simulink model "ScooterCharacteristic"  (R2024a)
settings: Solver=VariableStepAuto  StartTime=0.0  StopTime=Inf  RelTol=1e-3
libraries: fl_lib x6, nesl_utility x3
settings Model: Creator=vboutrou  LastModifiedBy=vboutrou
settings RTWCC: GPUComputeCapability=3.5
settings SimscapeCC: SimscapeLogType=all

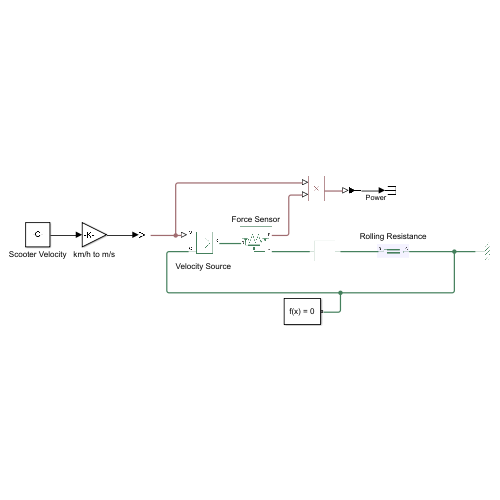
[thumbnail: Simulink's stored preview of the top-level diagram]
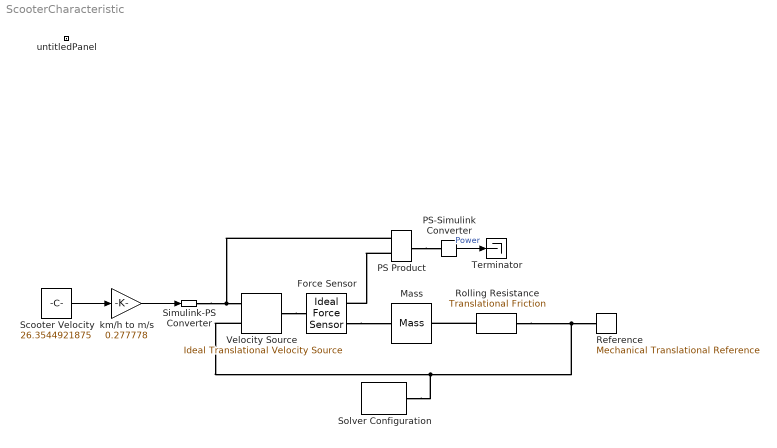
== system ScooterCharacteristic ==
  Force Sensor : fl_lib/Mechanical/Mechanical Sensors/Ideal Force Sensor
  Mass : fl_lib/Mechanical/Translational Elements/Mass  mass=90 kg  num_ports=foundation.enum.numPorts2.two  v_specify=off  v_priority=High  v=0 m/s  v_nominal_specify=off  v_nominal_value=1  v_nominal_unit=m/s  f_specify=off  f_priority=None  f=0 N  f_nominal_specify=off  f_nominal_value=1  f_nominal_unit=N
      settings: InternalSimscapePortConfiguration="{\"Bottom\":[],\"Left\":[{\"id\":\"M\",\"label\":\"\",\"type\":\"foundation.mechanical.translational.translational\"}],\"Right\":[{\"id\":\"N\",\"label\":\"\",\"type\":\"foundation.mechanical.translational.translational\"}],\"Top\":[]}"
  PS Product : fl_lib/Physical Signals/Functions/PS Product
  PS-Simulink Converter : nesl_utility/PS-Simulink Converter  PhysicalDomain=network_engine_domain  SubClassName=ps_output  LeftPortType=input  RightPortType=output  PseudoPeriodic=off  Frequencies=[]  VectorFormat=inherit  Unit=inherit  AffineConversion=off
  Reference : fl_lib/Mechanical/Translational Elements/Mechanical Translational Reference
  Rolling Resistance : fl_lib/Mechanical/Translational Elements/Translational Friction  brkwy_frc=20 N  brkwy_vel=0.1 m/s  Col_frc=14 N  visc_coef=3.1 N/(m/s)  v_specify=off  v_priority=None  v=0 m/s  v_nominal_specify=off  v_nominal_value=1  v_nominal_unit=m/s  f_specify=off  f_priority=None  f=0 N  f_nominal_specify=off  f_nominal_value=1  f_nominal_unit=N
      settings: InternalSimscapePortConfiguration="{\"Bottom\":[],\"Left\":[{\"id\":\"R\",\"label\":\"R\",\"type\":\"foundation.mechanical.translational.translational\"}],\"Right\":[{\"id\":\"C\",\"label\":\"C\",\"type\":\"foundation.mechanical.translational.translational\"}],\"Top\":[]}"
  Scooter Velocity : Constant  Value=26.3544921875
  Simulink-PS Converter : nesl_utility/Simulink-PS Converter  PhysicalDomain=network_engine_domain  SubClassName=ps_input  LeftPortType=input  RightPortType=output  PseudoPeriodic=off  Frequencies=[]  NoiseDistribution=none  NoiseParameters=[]  Unit=m/s  AffineConversion=off  FilteringAndDerivatives=provide  SimscapeFilterOrder=1  InputFilterTimeConstant=0.001  UdotUserProvided=0
  Solver Configuration : nesl_utility/Solver Configuration  PhysicalDomain=network_engine_domain  SubClassName=solver  LeftPortType=input  RightPortType=generic  Tones=[]  Harmonics=[]  SimulateNoise=off  Profile=off  UseLocalSampling=off  EnableSwitchedLinearOptims=on  FrequencyDomain=off  UseCCode=off  RelTol=0.001  AbsTol=0.001  MinStep=1e-09  ToWorkspace=off  RevertToSquareIcSolve=off  NumHomotopyIterations=100  PhasorMode=off  PhasorModeNumHarmonics=1  ConsistencySolver=NEWTON_XTOL_AFTER_FTOL  IndexReductionMethod=DerivativeReplacement  DoDC=on  ResidualTolerance=1e-09  ConsistencyTolSource=GLOBAL  ConsistencyAbsTol=0.001  ConsistencyRelTol=0.001  ConsistencyTolFactor=0.001  UseLocalSolver=off  LocalSolverChoice=NE_BACKWARD_EULER_ADVANCER  ResolveIndetEquations=on  FunctionEvalNumThread=1  LocalSolverSampleTime=0.001  DoFixedCost=off  MaxNonlinIter=3  MaxModeIter=2  ComputeImpulses=off  ImpulseIterations=2  LinearAlgebra=auto  LinearAlgebraNumThread=0  EquationFormulation=NE_TIME_EF  DelaysMemoryBudget=1024  AutomaticFiltering=on  FilteringTimeConstant=0.001  PartitionStorageMethod=AS_NEEDED  PartitionMemoryBudget=1024  PartitionMethod=ROBUST  MultibodyUseLocalSolver=off  MultibodyLocalSolverChoice=ODE1  MultibodyLocalSolverSampleTime=0.001
  Terminator : Terminator
  Velocity Source : fl_lib/Mechanical/Mechanical Sources/Ideal Translational Velocity Source
  km/h to m/s : Gain  Gain=0.277778
  untitledPanel : Subsystem  Tag=HiddenForWebPanel  IsWebBlockPanel=on
  wires:
  Scooter Velocity/1 -> km/h to m/s/1
  PS-Simulink Converter/1 -> Terminator/1  "Power"
  km/h to m/s/1 -> Simulink-PS Converter/1
  connections:
  Rolling Resistance/RConn1 -- Reference/LConn1 -- Velocity Source/RConn2 -- Solver Configuration/RConn1
  Force Sensor/RConn1 -- Mass/RConn1
  PS Product/LConn1 -- Simulink-PS Converter/RConn1 -- Velocity Source/RConn1
  Rolling Resistance/LConn1 -- Mass/LConn1
  Velocity Source/LConn1 -- Force Sensor/LConn1
  PS Product/LConn2 -- Force Sensor/RConn2
  PS Product/RConn1 -- PS-Simulink Converter/LConn1

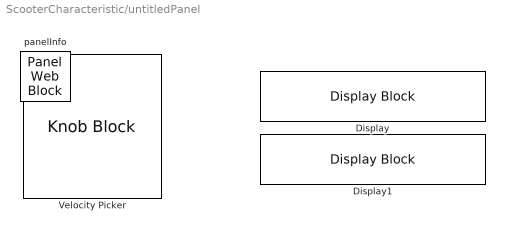
== system ScooterCharacteristic/untitledPanel ==
  Display : DisplayBlock  Tag=HiddenForWebPanel  PanelInfo="{\"height\":57,\"left\":184,\"panelId\":\"panelId-d0a485e7-f53d-4cca-bd4d-bce89a751458\",\"top\":83,\"type\":\"panelChild\",\"version\":\"2019b\",\"width\":252,\"zIndex\":1500006}"  LabelPosition=Hide  Format=Custom  Alignment=Left  Transparency=1  Layout=Fill available space  FormatString=Power: %3.1f W
  Display1 : DisplayBlock  Tag=HiddenForWebPanel  PanelInfo="{\"height\":57,\"left\":185,\"panelId\":\"panelId-d0a485e7-f53d-4cca-bd4d-bce89a751458\",\"top\":15,\"type\":\"panelChild\",\"version\":\"2019b\",\"width\":252,\"zIndex\":1500008}"  LabelPosition=Hide  Format=Custom  Alignment=Left  Transparency=1  Layout=Fill available space  FormatString=Velocity: %3.1f km/h
  Velocity Picker : KnobBlock  Tag=HiddenForWebPanel  PanelInfo="{\"height\":119,\"left\":20,\"panelId\":\"panelId-d0a485e7-f53d-4cca-bd4d-bce89a751458\",\"top\":21,\"type\":\"panelChild\",\"version\":\"2019b\",\"width\":154,\"zIndex\":1500002}"  LabelPosition=Bottom  ScaleMax=30  TickInterval=5
  panelInfo : PanelWebBlock  Tag=HiddenForWebPanel  PanelInfo="{\"compacted\":false,\"height\":159,\"isActiveTab\":true,\"labels\":{},\"left\":44,\"name\":\"Panel\",\"panelId\":\"panelId-d0a485e7-f53d-4cca-bd4d-bce89a751458\",\"tabIndex\":0,\"tabbedSetId\":\"tabbedSet6955295497\",\"top\":20,\"type\":\"panel\",\"version\":\"2019b\",\"visible\":true,\"width\":457,\"zIndex\":1500002}"  PanelSnapshot=<binary blob, 33744 chars, not shown>
